simulink model "caes_extraction_right_version"  (R2025b)
settings: Solver=VariableStepAuto  StopTime=3
settings Model: Creator=milenadaniltsenko  LastModifiedBy=milenadaniltsenko

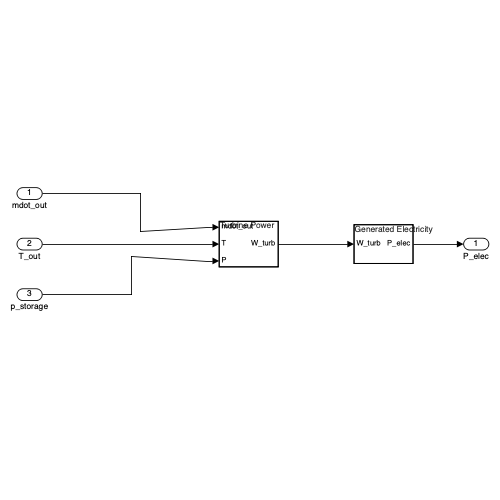
[thumbnail: Simulink's stored preview of the top-level diagram]
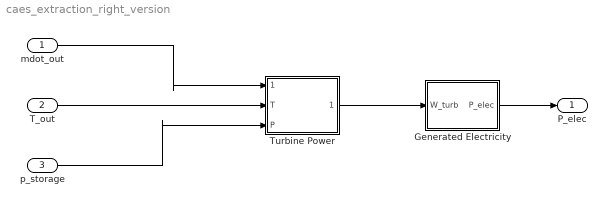
== system caes_extraction_right_version ==
  mdot_out : Inport
  T_out : Inport  Port=2
  p_storage : Inport  Port=3
  Generated Electricity : MATLAB Function  TreatAsAtomicUnit=on
  Turbine Power : MATLAB Function  TreatAsAtomicUnit=on
  P_elec : Outport
  wires:
  mdot_out/1 -> Turbine Power/1(mdot_out)
  Turbine Power/1(W_turb) -> Generated Electricity/1(W_turb)
  Generated Electricity/1(P_elec) -> P_elec/1
  T_out/1 -> Turbine Power/2(T)
  p_storage/1 -> Turbine Power/3(P)

== matlab function caes_extraction_right_version/Generated Electricity ==
  data: W_turb input; P_elec output
function P_elec = generator(W_turb)
    n_gen = 0.95; 
    P_elec = W_turb * n_gen;
end

== matlab function caes_extraction_right_version/Turbine Power ==
  data: mdot_out input; W_turb output; T input; P input
function W_turb = turbine(mdot_out, T, P)
    % Constants
    Cp = 1005;
    Patm = 101325;
    gamma = 1.4;
    n_turb = 0.8; %efficiency of the turbine

    if P <= Patm %if pressure is too low, then turbine does not generate power
        W_turb = 0;
    else
        % Isentropic expansion power formula
        expansion_ratio = (Patm / P)^((gamma - 1) / gamma);
        W_turb = mdot_out * Cp * T * n_turb * (1 - expansion_ratio);
    end
end
